simulink model "reciever"  (R2023a)
settings: Solver=FixedStepAuto  StartTime=0.0  StopTime=10.0  RelTol=1e-3
libraries: androidcommunicationlib x3, androidaudiovideolib x1
settings Model: Creator=Shesh  LastModifiedBy=Shesh
settings OptimizationCC: EnhancedBackFolding=on  PassReuseOutputArgsAs=Individual arguments  ZeroExternalMemoryAtStartup=off  ZeroInternalMemoryAtStartup=off  MaxStackSize=64  OptimizeBlockOrder=speed  DifferentSizesBufferReuse=on  OptimizationCustomize=off  EfficientTunableParamExpr=on
settings DebuggingCC: ParameterTunabilityLossMsg=error
settings HardwareCC: ProdBitPerPointer=32  ProdBitPerSizeT=32  ProdBitPerPtrDiffT=32  ProdLargestAtomicInteger=Long  ProdLargestAtomicFloat=Double  ProdWordSize=32  ProdHWDeviceType=ARM Compatible->ARM Cortex
settings SFSimCC: MATLABDynamicMemAlloc=off
settings RTWCC: Description=Embedded Coder  SystemTargetFile=ert.tlc  HardwareBoard=Android Device  TLCOptions="-aInlineSetEventsForThisBaseRateFcn=TLC_FALSE -aSuppressMultiTaskScheduler=TLC_FALSE  -aRateBasedStepFcn=0"  TemplateMakefile=ert_default_tmf  RTWVerbose=off  Toolchain=Android SDK/NDK Tools
settings CodeAppCC: ForceParamTrailComments=on  IgnoreCustomStorageClasses=off  OperatorAnnotations=on  SimulinkDataObjDesc=on  SFDataObjDesc=on  InsertBlockDesc=on

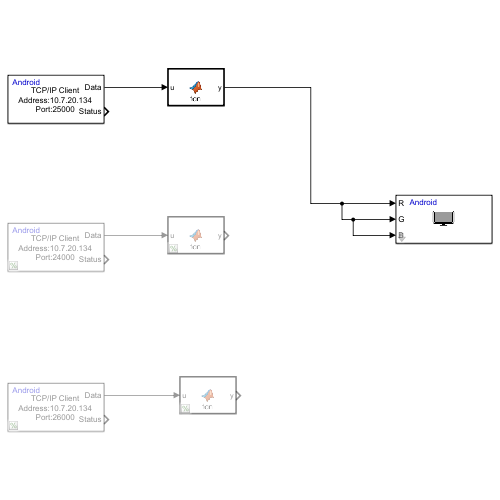
[thumbnail: Simulink's stored preview of the top-level diagram]
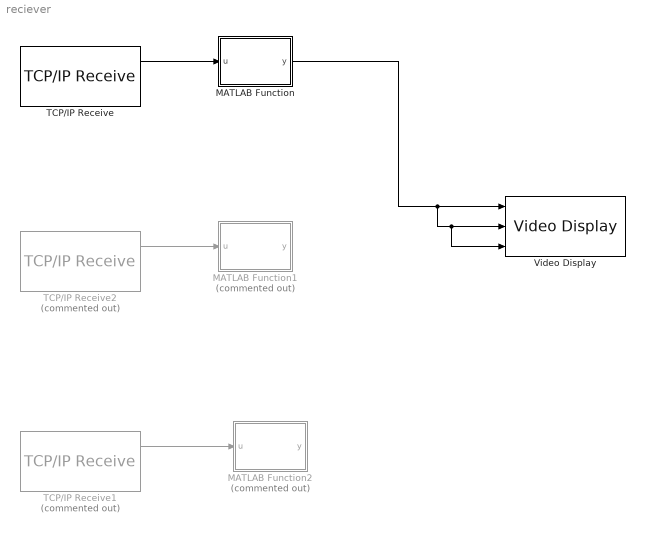
== system reciever ==
  MATLAB Function : MATLAB Function  TreatAsAtomicUnit=on
  MATLAB Function1 : MATLAB Function  Commented=on  TreatAsAtomicUnit=on
  MATLAB Function2 : MATLAB Function  Commented=on  TreatAsAtomicUnit=on
  TCP/IP Receive : androidcommunicationlib/TCP//IP Receive  TCPReceiveId=untitled1/TCP//IP_Receive  Mode_=Client  LocalServerPort_=25000  RemoteAddr_=10.7.20.134  RemoteServerPort_=25000  DataType_=uint8  DataSize_=25344  SampleTime_=0.1  ClientPortBindingSelection_=off  ClientPortToBind_=35000  BlockingMode_=off  BlockTimeout_=0.1
  TCP/IP Receive1 : androidcommunicationlib/TCP//IP Receive  Commented=on  TCPReceiveId=untitled1/TCP//IP_Receive1  Mode_=Client  LocalServerPort_=25000  RemoteAddr_=10.7.20.134  RemoteServerPort_=26000  DataType_=uint8  DataSize_=25344  SampleTime_=0.1  ClientPortBindingSelection_=off  ClientPortToBind_=35000  BlockingMode_=off  BlockTimeout_=0.1
  TCP/IP Receive2 : androidcommunicationlib/TCP//IP Receive  Commented=on  TCPReceiveId=untitled1/TCP//IP_Receive2  Mode_=Client  LocalServerPort_=25000  RemoteAddr_=10.7.20.134  RemoteServerPort_=24000  DataType_=uint8  DataSize_=25344  SampleTime_=0.1  ClientPortBindingSelection_=off  ClientPortToBind_=35000  BlockingMode_=off  BlockTimeout_=0.1
  Video Display : androidaudiovideolib/Video Display  BlockPlatform=Android
  wires:
  TCP/IP Receive/1 -> MATLAB Function/1(u)
  TCP/IP Receive2/1 -> MATLAB Function1/1(u)
  TCP/IP Receive1/1 -> MATLAB Function2/1(u)
  MATLAB Function/1(y) -> Video Display/3, Video Display/2, Video Display/1

== matlab function reciever/MATLAB Function ==
  data: u input; y output
function y = fcn(u)
    u = reshape(u,176,144);
y = u;

== matlab function reciever/MATLAB Function2 ==
  data: u input; y output
function y = fcn(u)
    u = reshape(u,176,144);
y = u;

== matlab function reciever/MATLAB Function1 ==
  data: u input; y output
function y = fcn(u)
    u = reshape(u,176,144);
y = u;
